simulink model "CSTR_PI"  (R2021b)
settings: Solver=FixedStepAuto  StartTime=0  StopTime=45  FixedStep=Ts  RelTol=1e-3  EnableMultiTasking=on
PreLoadFcn:
  | Ts = 0.5;
  | load cstr_data.mat
values from neighbouring files (symbols this model uses):
  a_vec = [0.384207621232 0.492686723525 0.580956543032 0.649017079753 0.696868333688 0.724510304838 0.731942993202 0.71916639878 0.686180521572 0.632985361578 0.559580918799 0.465967193234 ... (15 elements, 15x1)]    [gains.mat]    (also in settings.mat)
  b_vec = [0.0628087670629 0.0875474545058 0.110088960049 0.130433283691 0.148580425434 0.164530385276 0.178283163218 0.18983875926 0.199197173402 0.206358405644 0.211322455985 0.214089324427 ... (15 elements, 15x1)]    [gains.mat]    (also in settings.mat)
  conc_noise = 0    [init_vars.m]    (also in run_PI.m = abs(CrEQ(1)-CrEQ(5)) * noise / 100.0; run_benchmark.m = abs(CrEQ(1)-CrEQ(5))*noise_magnitude; run_brain.m = abs(CrEQ(1)-CrEQ(5))*noise/100.0)
  Cr_vec = [2:.5:9]    [init_vars.m]
  Cref_signal = 2    [init_vars.m]
  CrEQ = [8.57 6.9275 5.285 3.6425 2]    [equilibrium.mat]    (also in settings.mat)
  Ki_vec = [-7.985128543 -6.23612330817 -4.75246287755 -3.53414725114 -2.58117642895 -1.89355041096 -1.47126919718 -1.31433278761 -1.42274118225 -1.7964943811 -2.43559238416 -3.34003519143 ... (15 elements, 15x1)]    [gains.mat]    (also in settings.mat)
  Kp_vec = [-2.00046148742 -2.31845608468 -2.65393524902 -3.00689898043 -3.37734727893 -3.76528014451 -4.17069757716 -4.5935995769 -5.03398614371 -5.49185727761 -5.96721297858 -6.46005324663 ... (15 elements, 15x1)]    [gains.mat]    (also in settings.mat)
  Kt_vec = [3.60620000482 3.57285570623 3.55992955218 3.56742154268 3.59533167773 3.64365995732 3.71240638145 3.80157095013 3.91115366335 4.04115452112 4.19157352344 4.3624106703 ... (15 elements, 15x1)]    [gains.mat]    (also in settings.mat)
  TcEQ = [297.97975414 305.238623843 296.793917779 290.535352357 305.034880275]    [equilibrium.mat]    (also in settings.mat)
  temp_noise = 0    [init_vars.m]    (also in run_PI.m = abs(TrEQ(1)-TrEQ(5)) * noise / 100.0; run_benchmark.m = abs(TrEQ(1)-TrEQ(5))*noise_magnitude; run_brain.m = abs(TrEQ(1)-TrEQ(5))*noise/100.0)
  TrEQ = [311.261174032 327.996759348 341.108442564 354.724619775 373.131126217]    [equilibrium.mat]    (also in settings.mat)
undefined symbols (not defined in the file or in its folder): DiscIntNeverNeededParam, sigbuilder_block
settings Model: Creator=The MathWorks, Inc.  LastModifiedBy=scott
settings SolverCC: AlgebraicLoopSolver=TrustRegion
settings DataIOCC: InitialState=[311.267; 8.5695]  LimitDataPoints=on  SaveFormat=Array  ReturnWorkspaceOutputs=off  SignalLoggingName=logsOut
settings OptimizationCC: BooleanDataType=off  DefaultParameterBehavior=Inlined  InlineInvariantSignals=on  BufferReuse=off  ExpressionDepthLimit=2147483647  InitFltsAndDblsToZero=on  LifeSpan=inf
settings DebuggingCC: SaveWithParameterizedLinksMsg=none  UnderspecifiedInitializationDetection=Classic  MergeDetectMultiDrivingBlocksExec=none  CheckExecutionContextPreStartOutputMsg=on  SignalResolutionControl=TryResolveAllWithWarning  MultiTaskDSMMsg=warning  MultiTaskCondExecSysMsg=none  AllowSymbolicDim=off  StateNameClashWarn=warning  SFUnexpectedBacktrackingDiag=warning  SFNoUnconditionalDefaultTransitionDiag=warning  SFExecutionAtInitializationDiag=none  SFMachineParentedDataDiag=warning  ArithmeticOperatorsInVariantConditions=warning
settings HardwareCC: ProdBitPerPointer=32  ProdBitPerSizeT=32  ProdBitPerPtrDiffT=32  ProdLargestAtomicFloat=None  ProdIntDivRoundTo=Undefined  ProdEndianess=Unspecified  ProdWordSize=32  ProdHWDeviceType=32-bit Generic  TargetUnknown=on
settings ModelReferenceCC: PropagateSignalLabelsOutOfModel=off
settings SFSimCC: SimUseLocalCustomCode=off  CustomCodeUndefinedFunction=UseInterfaceOnly
settings RTWCC: RTWUseLocalCustomCode=off
settings CodeAppCC: StateflowObjectComments=on
settings GRTTargetCC: TargetFcnLib=ansi_tfl_tmw.mat  TargetLangStandard=C89/C90 (ANSI)  CombineOutputUpdateFcns=off  GRTInterface=on
settings ConfigComp: CovMetricSettings=dw  CovSaveCumulativeToWorkspaceVar=on  CovSaveSingleToWorkspaceVar=on  CovExternalEMLEnable=off  CovSFcnEnable=off

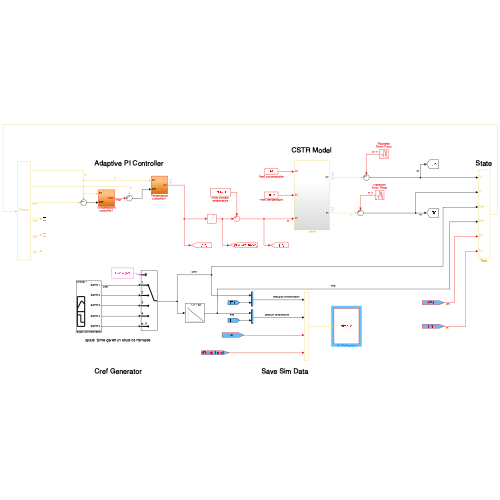
[thumbnail: Simulink's stored preview of the top-level diagram]
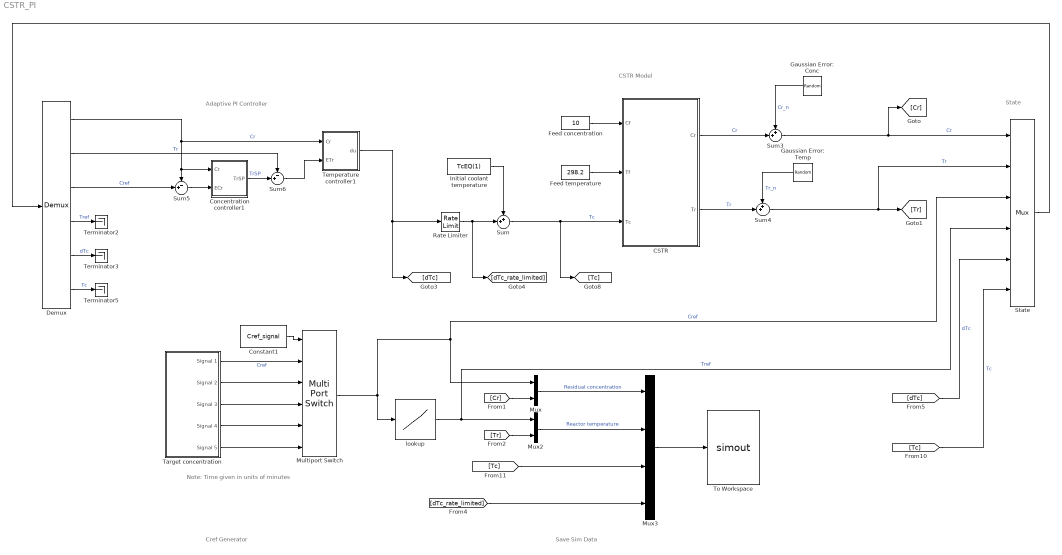
== system CSTR_PI ==
  note: Note: Time given in units of minutes
  note: Adaptive PI Controller
  note: CSTR Model
  note: Cref Generator
  note: State
  note: Save Sim Data
  CSTR : Subsystem
  Concentration controller1 : Subsystem
  Constant1 : Constant  Value=Cref_signal
  Demux : Demux  Outputs=6
      settings: DisplayOption=none
  Feed concentration : Constant  Value=10  SampleTime=0
  Feed temperature : Constant  Value=298.2  SampleTime=0
  Gaussian Error: Conc : RandomNumber  Variance=conc_noise*conc_noise  Seed=randi(100)  SampleTime=Ts
  Gaussian Error: Temp : RandomNumber  Variance=temp_noise*temp_noise  Seed=randi(100)  SampleTime=Ts
  Initial coolant temperature : Constant  Value=TcEQ(1)  SampleTime=0
  Multiport Switch : MultiPortSwitch  Inputs=5
  Mux : Mux  Inputs=2
  Mux2 : Mux  Inputs=2
  Mux3 : Mux
  Rate Limiter : RateLimiter  RisingSlewLimit=10  FallingSlewLimit=-10  SampleTimeMode=inherited
  State : Mux  Inputs=6
      settings: DisplayOption=signals
  Sum : Sum  Inputs=++|
  Sum3 : Sum  Inputs=++|
  Sum4 : Sum  Inputs=++|
  Sum5 : Sum  Inputs=-+|
  Sum6 : Sum  Inputs=-+|
  Target concentration : Subsystem  Tag=STV Subsys  LoadFcn=sigbuilder_block('load');  StartFcn=sigbuilder_block('start');  StopFcn=sigbuilder_block('stop');  ClipboardFcn=sigbuilder_block('clipboard');  mask(Sigbuilder block){tuvar=[0:10]}
      mask help: Simulink:masks:SigbuilderBlock_MD
      mask init:
      | if ~strcmp(get_param(bdroot(gcbh),'SimulationStatus'),'stopped') tuvar = sigbuilder_block('maskInit'); end
      settings: CopyFcn=sigbuilder_block('copy');  DeleteFcn=sigbuilder_block('delete');  ModelCloseFcn=sigbuilder_block('modelClose');  PreSaveFcn=sigbuilder_block('preSave');  PauseFcn=sigbuilder_block('pause');  ContinueFcn=sigbuilder_block('continue');  NameChangeFcn=sigbuilder_block('namechange');  OpenFcn=sigbuilder_block('open',[661 266 1131 668 ]);  CloseFcn=sigbuilder_block('close');
      mask Display: plot(0, 0, 100, 100,[2, 2, 32, 32, 2], [68, 8, 8, 68, 68],[32, 2], [38, 38], [32, 19, 2],[53, 60, 44], [32, 17, 17, 2],[16, 16, 31, 31]);txt = getActiveGroup(gcbh);text(2, 100, txt,'verticalAlignment', 'top');
  Temperature controller1 : Subsystem
  Terminator2 : Terminator
  Terminator3 : Terminator
  Terminator5 : Terminator
  To Workspace : ToWorkspace  VariableName=simout  SampleTime=-1
  lookup : Lookup_n-D  NumberOfTableDimensions=1  LookupTableObject=''  BreakpointsForDimension1=flipud(CrEQ)  Table=flipud(TrEQ)  RndMeth=Simplest  InputSameDT=on
  wires:
  Feed concentration/1 -> CSTR/1(Cf)
  Feed temperature/1 -> CSTR/2(Tf)
  Initial coolant temperature/1 -> Sum/1
  [Cr] -> Mux/2
  Mux2/1 -> Mux3/2  "Reactor temperature"
  Mux/1 -> Mux3/1  "Residual concentration"
  [dTc_rate_limited] -> Mux3/4
  [Tr] -> Mux2/2
  lookup/1 -> State/4, Mux2/1  "Tref"
  Sum/1 -> CSTR/3(Tc), [Tc]  "Tc"
  Mux3/1 -> To Workspace/1
  Rate Limiter/1 -> Sum/2, [dTc_rate_limited]
  Constant1/1 -> Multiport Switch/1
  Target concentration/1(Signal 1) -> Multiport Switch/2  "Cref"
  Target concentration/4(Signal 4) -> Multiport Switch/5
  Target concentration/2(Signal 2) -> Multiport Switch/3
  Target concentration/3(Signal 3) -> Multiport Switch/4
  [dTc] -> State/5  "dTc"
  CSTR/1(Cr) -> Sum3/2  "Cr"
  Gaussian Error: Conc/1 -> Sum3/1  "Cr_n"
  Gaussian Error: Temp/1 -> Sum4/1  "Tr_n"
  Temperature controller1/1(du) -> [dTc], Rate Limiter/1
  [Tc] -> State/6  "Tc"
  [Tc] -> Mux3/3
  CSTR/2(Tr) -> Sum4/2  "Tr"
  Sum3/1 -> [Cr], State/1  "Cr"
  Sum4/1 -> [Tr], State/2  "Tr"
  Multiport Switch/1 -> State/3, Mux/1, lookup/1  "Cref"
  Demux/3 -> Sum5/2  "Cref"
  Demux/1 -> Concentration controller1/1(Cr), Sum5/1, Temperature controller1/1(Cr)  "Cr"
  Demux/5 -> Terminator3/1  "dTc"
  Sum5/1 -> Concentration controller1/2(ECr)
  Demux/6 -> Terminator5/1  "Tc"
  Demux/2 -> Sum6/1  "Tr"
  Demux/4 -> Terminator2/1  "Tref"
  Concentration controller1/1(TrSP) -> Sum6/2  "TrSP"
  State/1 -> Demux/1
  Sum6/1 -> Temperature controller1/2(ETr)
  Target concentration/5(Signal 5) -> Multiport Switch/6

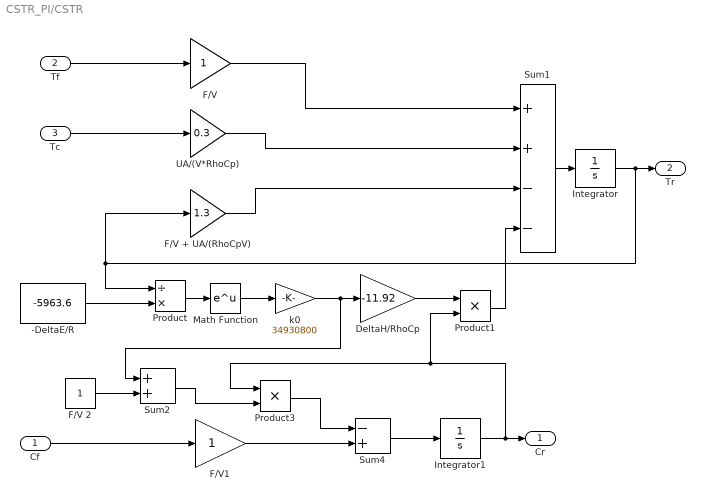
== system CSTR_PI/CSTR ==
  Cf : Inport
  Tf : Inport  Port=2
  Tc : Inport  Port=3
  -DeltaE/R : Constant  Value=-5963.6  SampleTime=0
  DeltaH/RhoCp : Gain  Gain=-11.92  SaturateOnIntegerOverflow=on  OutDataTypeStr=Inherit: Same as input  ParamDataTypeStr=Inherit: Same as input
  F/V : Gain  SaturateOnIntegerOverflow=on  OutDataTypeStr=Inherit: Same as input  ParamDataTypeStr=Inherit: Same as input
  F/V + UA/(RhoCpV) : Gain  Gain=1.3  SaturateOnIntegerOverflow=on  OutDataTypeStr=Inherit: Same as input  ParamDataTypeStr=Inherit: Same as input
  F/V 2 : Constant  SampleTime=0
  F/V1 : Gain  SaturateOnIntegerOverflow=on  OutDataTypeStr=Inherit: Same as input  ParamDataTypeStr=Inherit: Same as input
  Integrator : Integrator  InitialCondition=TrEQ(1)  LimitOutput=on  LowerSaturationLimit=0
  Integrator1 : Integrator  InitialCondition=CrEQ(1)  LimitOutput=on  LowerSaturationLimit=0
  Math Function : Math  SignedPower=on  SaturateOnIntegerOverflow=on
  Product : Product  Inputs=/*  InputSameDT=on  RndMeth=Zero  SaturateOnIntegerOverflow=on  OutDataTypeStr=Inherit: Same as first input
  Product1 : Product  InputSameDT=on  RndMeth=Zero  SaturateOnIntegerOverflow=on  OutDataTypeStr=Inherit: Same as first input
  Product3 : Product  InputSameDT=on  RndMeth=Zero  SaturateOnIntegerOverflow=on  OutDataTypeStr=Inherit: Same as first input
  Sum1 : Sum  Inputs=++--  InputSameDT=on  SaturateOnIntegerOverflow=on  OutDataTypeStr=Inherit: Same as first input
  Sum2 : Sum  InputSameDT=on  SaturateOnIntegerOverflow=on  OutDataTypeStr=Inherit: Same as first input
  Sum4 : Sum  Inputs=-+  InputSameDT=on  SaturateOnIntegerOverflow=on  OutDataTypeStr=Inherit: Same as first input
  UA/(V*RhoCp) : Gain  Gain=0.3  SaturateOnIntegerOverflow=on  OutDataTypeStr=Inherit: Same as input  ParamDataTypeStr=Inherit: Same as input
  k0 : Gain  Gain=34930800  SaturateOnIntegerOverflow=on  OutDataTypeStr=Inherit: Same as input  ParamDataTypeStr=Inherit: Same as input
  Cr : Outport
  Tr : Outport  Port=2
  wires:
  F/V/1 -> Sum1/1
  Sum1/1 -> Integrator/1
  Integrator/1 -> Product/1, F/V + UA/(RhoCpV)/1, Tr/1
  UA/(V*RhoCp)/1 -> Sum1/2
  F/V + UA/(RhoCpV)/1 -> Sum1/3
  Product/1 -> Math Function/1
  Math Function/1 -> k0/1
  DeltaH/RhoCp/1 -> Product1/1
  Product1/1 -> Sum1/4
  k0/1 -> DeltaH/RhoCp/1, Sum2/1
  -DeltaE/R/1 -> Product/2
  Product3/1 -> Sum4/1
  Sum4/1 -> Integrator1/1
  Integrator1/1 -> Product1/2, Product3/1, Cr/1
  F/V 2/1 -> Sum2/2
  F/V1/1 -> Sum4/2
  Tf/1 -> F/V/1
  Cf/1 -> F/V1/1
  Tc/1 -> UA/(V*RhoCp)/1
  Sum2/1 -> Product3/2

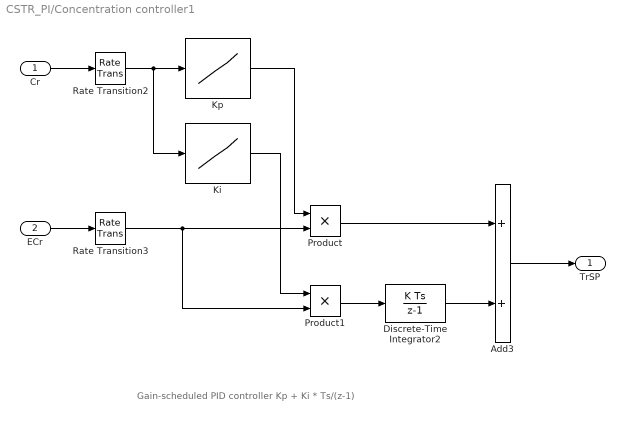
== system CSTR_PI/Concentration controller1 ==
  note: Gain-scheduled PID controller Kp + Ki * Ts/(z-1)
  Cr : Inport
  ECr : Inport  Port=2
  Add3 : Sum
  Discrete-Time Integrator2 : DiscreteIntegrator  InitialCondition=TrEQ(1)  SampleTime=Ts  ICPrevOutput=DiscIntNeverNeededParam  ICPrevScaledInput=DiscIntNeverNeededParam
  Ki : Lookup_n-D  NumberOfTableDimensions=1  LookupTableObject=''  BreakpointsForDimension1=Cr_vec  Table=Ki_vec  InternalRulePriority=Speed  RndMeth=Simplest  InputSameDT=on
  Kp : Lookup_n-D  NumberOfTableDimensions=1  LookupTableObject=''  BreakpointsForDimension1=Cr_vec  Table=Kp_vec  InternalRulePriority=Speed  RndMeth=Simplest  InputSameDT=on
  Product : Product
  Product1 : Product
  Rate Transition2 : RateTransition  OutPortSampleTime=Ts
  Rate Transition3 : RateTransition  OutPortSampleTime=Ts
  TrSP : Outport
  wires:
  ECr/1 -> Rate Transition3/1
  Discrete-Time Integrator2/1 -> Add3/2
  Product/1 -> Add3/1
  Add3/1 -> TrSP/1
  Cr/1 -> Rate Transition2/1
  Kp/1 -> Product/1
  Rate Transition2/1 -> Ki/1, Kp/1
  Product1/1 -> Discrete-Time Integrator2/1
  Rate Transition3/1 -> Product1/2, Product/2
  Ki/1 -> Product1/1

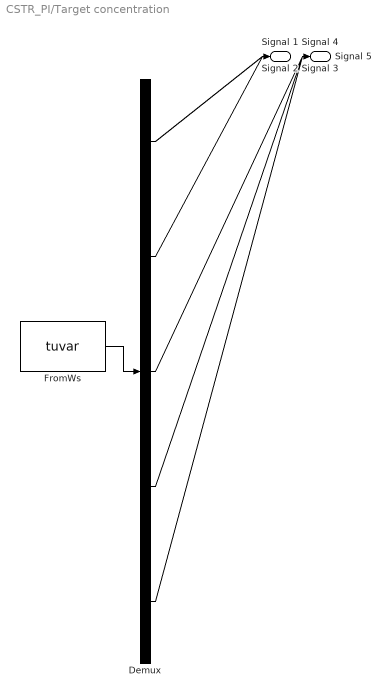
== system CSTR_PI/Target concentration ==
  Demux : Demux  Tag=STV Demux  Outputs=5
      settings: DisplayOption=none
  FromWs : FromWorkspace  Tag=STV FromWs  VariableName=tuvar
      SigBuilderData=|
      | common.afterFinalStr = 'Extrapolate'
      | common.sampleTime = 0
      | dataSet.timeRange = [0 90]
      | dataSet.name = 'Group 1'
      | sbobj.Groups.Name = 'Group 1'
      | sbobj.Groups.Signals(1).Name = 'Signal 1'
      | sbobj.Groups.Signals(1).XData = [0 26 90]
      | sbobj.Groups.Signals(1).YData = [8.57 2 2]
      | sbobj.Groups.Signals(2).Name = 'Signal 2'
      | sbobj.Groups.Signals(2).XData = [0 10 36 90]
      | sbobj.Groups.Signals(2).YData = [8.57 8.57 2 2]
      | sbobj.Groups.Signals(3).Name = 'Signal 3'
      | sbobj.Groups.Signals(3).XData = [0 20 46 90]
      | sbobj.Groups.Signals(3).YData = [8.57 8.57 2 2]
      | sbobj.Groups.Signals(4).Name = 'Signal 4'
      | sbobj.Groups.Signals(4).XData = [0 30 56 90]
      | sbobj.Groups.Signals(4).YData = [9.57 9.57 2 2]
      | sbobj.Groups.Signals(5).Name = 'Signal 5'
      | sbobj.Groups.Signals(5).XData = [0 90]
      | sbobj.Groups.Signals(5).YData = [8.57 8.57]
      | sbobj.Groups.TimeRange = [0 90]
  Signal 1 : Outport  Tag=STV Outport
  Signal 2 : Outport  Tag=STV Outport  Port=2
  Signal 3 : Outport  Tag=STV Outport  Port=3
  Signal 4 : Outport  Tag=STV Outport  Port=4
  Signal 5 : Outport  Tag=STV Outport  Port=5
  wires:
  FromWs/1 -> Demux/1
  Demux/1 -> Signal 1/1
  Demux/2 -> Signal 2/1
  Demux/3 -> Signal 3/1
  Demux/4 -> Signal 4/1
  Demux/5 -> Signal 5/1

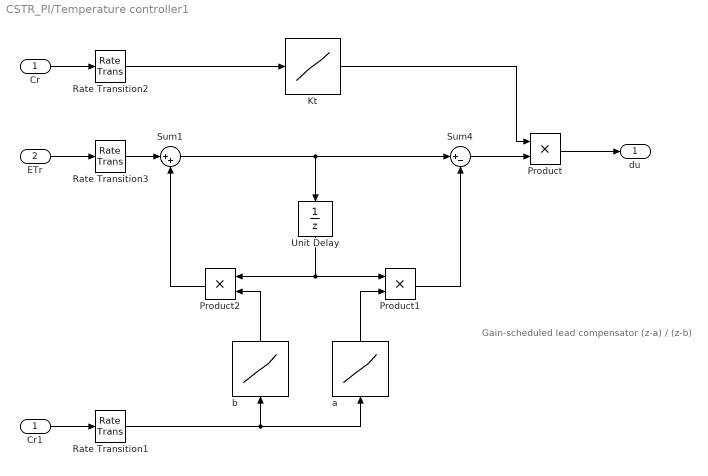
== system CSTR_PI/Temperature controller1 ==
  note: Gain-scheduled lead compensator
      | (z-a) / (z-b)
  Cr : Inport
  ETr : Inport  Port=2
  Cr1 : InportShadow
  Kt : Lookup_n-D  NumberOfTableDimensions=1  LookupTableObject=''  BreakpointsForDimension1=Cr_vec  Table=Kt_vec  InternalRulePriority=Speed  RndMeth=Simplest  InputSameDT=on
  Product : Product
  Product1 : Product
  Product2 : Product
  Rate Transition1 : RateTransition  OutPortSampleTime=Ts
  Rate Transition2 : RateTransition  OutPortSampleTime=Ts
  Rate Transition3 : RateTransition  OutPortSampleTime=Ts
  Sum1 : Sum  Inputs=|++
  Sum4 : Sum  Inputs=|+-
  Unit Delay : UnitDelay  SampleTime=Ts  HasFrameUpgradeWarning=on
  a : Lookup_n-D  NumberOfTableDimensions=1  LookupTableObject=''  BreakpointsForDimension1=Cr_vec  Table=a_vec  InternalRulePriority=Speed  RndMeth=Simplest  InputSameDT=on
  b : Lookup_n-D  NumberOfTableDimensions=1  LookupTableObject=''  BreakpointsForDimension1=Cr_vec  Table=b_vec  InternalRulePriority=Speed  RndMeth=Simplest  InputSameDT=on
  du : Outport
  wires:
  Product/1 -> du/1
  Product1/1 -> Sum4/2
  Sum1/1 -> Sum4/1, Unit Delay/1
  Sum4/1 -> Product/2
  Product2/1 -> Sum1/2
  Unit Delay/1 -> Product1/1, Product2/1
  ETr/1 -> Rate Transition3/1
  Rate Transition3/1 -> Sum1/1
  Cr/1 -> Rate Transition2/1
  Rate Transition2/1 -> Kt/1
  Kt/1 -> Product/1
  Cr1/1 -> Rate Transition1/1
  a/1 -> Product1/2
  Rate Transition1/1 -> b/1, a/1
  b/1 -> Product2/2
